simulink model "soft_finger_main"  (R2022b)
settings: Solver=VariableStepAuto  StartTime=0.0  StopTime=50  RelTol=1e-3
undefined symbols (not defined in the file): bounds, cf, D, DiscIntNeverNeededParam, Discrete, Fingertip, forceSetPoint, K, M, mylib, rho, sensor_locs, Time, X, Y, Z
libraries: sm_lib x117, nesl_utility x97, fl_lib x81, ee_lib x6, simulink x4, statsLibrary x3, slpidlib x2, deeplib x1, ctrlSharedLib x1
(part 2 of 5)

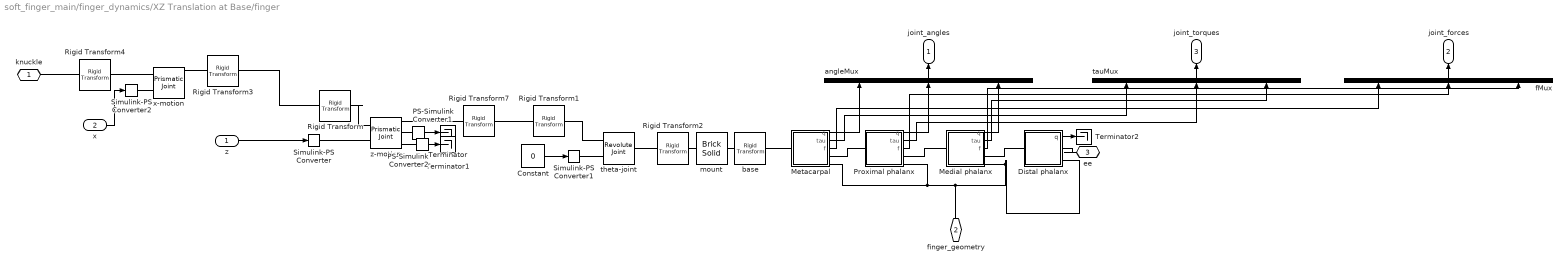
== system soft_finger_main/finger_dynamics/XZ Translation at Base/finger ==
  z : Inport
  x : Inport  Port=2
  Constant : Constant  Value=0
  Distal phalanx : Subsystem  mask{D=D, L=15, K=K, M=M, rho=rho, mu=1, muV=1}
  Medial phalanx : Subsystem  mask{D=D, L=24, K=K, M=M, rho=rho, mu=1, muV=1}
  Metacarpal : Subsystem  mask{D=D, L=64, K=K, M=M, rho=rho, mu=1, muV=1}
  PS-Simulink Converter1 : nesl_utility/PS-Simulink Converter  PhysicalDomain=network_engine_domain  SubClassName=ps_output  LeftPortType=input  RightPortType=output  PseudoPeriodic=off  Frequencies=[]  VectorFormat=1-D array  Unit=inherit  AffineConversion=off
  PS-Simulink Converter2 : nesl_utility/PS-Simulink Converter  PhysicalDomain=network_engine_domain  SubClassName=ps_output  LeftPortType=input  RightPortType=output  PseudoPeriodic=off  Frequencies=[]  VectorFormat=1-D array  Unit=inherit  AffineConversion=off
  Proximal phalanx : Subsystem  mask{D=D, L=39, K=K, M=M, rho=rho, mu=1, muV=1}
  Rigid Transform : sm_lib/Frames and Transforms/Rigid Transform  TranslationMethod=Cartesian  TranslationStandardOffset=40  TranslationLengthUnit=mm  TranslationStandardAxis=+Z  TranslationCartesianOffset=initPos  TranslationROffset=0  TranslationROffsetUnits=m  TranslationZOffset=0  TranslationZOffsetUnits=m  TranslationThetaOffset=0  TranslationThetaOffsetUnits=deg  RotationMethod=StandardAxis  RotationAngleUnits=deg  RotationStandardAxis=+Z  RotationAngle=180  RotationArbitraryAxis=[0 0 1]  FollAlignAxisA=+X  BaseAlignAxisA=+Y  FollAlignAxisB=+Y  BaseAlignAxisB=+Z  RotationSequenceAxes=FollowerAxes  RotationSequence=XYX  RotationSequenceAngles=[0 0 0]  RotationSequenceAnglesUnits=deg  RotationMatrix=[1 0 0; 0 1 0; 0 0 1]  Quaternion=[1 0 0 0]
  Rigid Transform1 : sm_lib/Frames and Transforms/Rigid Transform  TranslationMethod=None  TranslationStandardOffset=0  TranslationLengthUnit=m  TranslationStandardAxis=+Z  TranslationCartesianOffset=[0 0 0]  TranslationROffset=0  TranslationROffsetUnits=m  TranslationZOffset=0  TranslationZOffsetUnits=m  TranslationThetaOffset=0  TranslationThetaOffsetUnits=deg  RotationMethod=StandardAxis  RotationAngleUnits=deg  RotationStandardAxis=-X  RotationAngle=90  RotationArbitraryAxis=[0 0 1]  FollAlignAxisA=+X  BaseAlignAxisA=+Y  FollAlignAxisB=+Y  BaseAlignAxisB=+Z  RotationSequenceAxes=FollowerAxes  RotationSequence=XYX  RotationSequenceAngles=[0 0 0]  RotationSequenceAnglesUnits=deg  RotationMatrix=[1 0 0; 0 1 0; 0 0 1]  Quaternion=[1 0 0 0]
  Rigid Transform2 : sm_lib/Frames and Transforms/Rigid Transform  TranslationMethod=None  TranslationStandardOffset=0  TranslationLengthUnit=m  TranslationStandardAxis=+Z  TranslationCartesianOffset=[0 0 0]  TranslationROffset=0  TranslationROffsetUnits=m  TranslationZOffset=0  TranslationZOffsetUnits=m  TranslationThetaOffset=0  TranslationThetaOffsetUnits=deg  RotationMethod=StandardAxis  RotationAngleUnits=deg  RotationStandardAxis=-X  RotationAngle=90  RotationArbitraryAxis=[0 0 1]  FollAlignAxisA=+X  BaseAlignAxisA=+Y  FollAlignAxisB=+Y  BaseAlignAxisB=+Z  RotationSequenceAxes=FollowerAxes  RotationSequence=XYX  RotationSequenceAngles=[0 0 0]  RotationSequenceAnglesUnits=deg  RotationMatrix=[1 0 0; 0 1 0; 0 0 1]  Quaternion=[1 0 0 0]
  Rigid Transform3 : sm_lib/Frames and Transforms/Rigid Transform  TranslationMethod=None  TranslationStandardOffset=0  TranslationLengthUnit=m  TranslationStandardAxis=+Z  TranslationCartesianOffset=[0 0 0]  TranslationROffset=0  TranslationROffsetUnits=m  TranslationZOffset=0  TranslationZOffsetUnits=m  TranslationThetaOffset=0  TranslationThetaOffsetUnits=deg  RotationMethod=StandardAxis  RotationAngleUnits=deg  RotationStandardAxis=+Y  RotationAngle=90  RotationArbitraryAxis=[0 0 1]  FollAlignAxisA=+X  BaseAlignAxisA=+Y  FollAlignAxisB=+Y  BaseAlignAxisB=+Z  RotationSequenceAxes=FollowerAxes  RotationSequence=XYX  RotationSequenceAngles=[0 0 0]  RotationSequenceAnglesUnits=deg  RotationMatrix=[1 0 0; 0 1 0; 0 0 1]  Quaternion=[1 0 0 0]
  Rigid Transform4 : sm_lib/Frames and Transforms/Rigid Transform  TranslationMethod=None  TranslationStandardOffset=0  TranslationLengthUnit=m  TranslationStandardAxis=+Z  TranslationCartesianOffset=[0 0 0]  TranslationROffset=0  TranslationROffsetUnits=m  TranslationZOffset=0  TranslationZOffsetUnits=m  TranslationThetaOffset=0  TranslationThetaOffsetUnits=deg  RotationMethod=StandardAxis  RotationAngleUnits=deg  RotationStandardAxis=-Y  RotationAngle=90  RotationArbitraryAxis=[0 0 1]  FollAlignAxisA=+X  BaseAlignAxisA=+Y  FollAlignAxisB=+Y  BaseAlignAxisB=+Z  RotationSequenceAxes=FollowerAxes  RotationSequence=XYX  RotationSequenceAngles=[0 0 0]  RotationSequenceAnglesUnits=deg  RotationMatrix=[1 0 0; 0 1 0; 0 0 1]  Quaternion=[1 0 0 0]
  Rigid Transform7 : sm_lib/Frames and Transforms/Rigid Transform  TranslationMethod=None  TranslationStandardOffset=0  TranslationLengthUnit=m  TranslationStandardAxis=+Z  TranslationCartesianOffset=[0 0 0]  TranslationROffset=0  TranslationROffsetUnits=m  TranslationZOffset=0  TranslationZOffsetUnits=m  TranslationThetaOffset=0  TranslationThetaOffsetUnits=deg  RotationMethod=StandardAxis  RotationAngleUnits=rad  RotationStandardAxis=+Y  RotationAngle=0  RotationArbitraryAxis=[0 0 1]  FollAlignAxisA=+X  BaseAlignAxisA=+Y  FollAlignAxisB=+Y  BaseAlignAxisB=+Z  RotationSequenceAxes=FollowerAxes  RotationSequence=XYX  RotationSequenceAngles=[0 0 0]  RotationSequenceAnglesUnits=deg  RotationMatrix=[1 0 0; 0 1 0; 0 0 1]  Quaternion=[1 0 0 0]
  Simulink-PS Converter : nesl_utility/Simulink-PS Converter  PhysicalDomain=network_engine_domain  SubClassName=ps_input  LeftPortType=input  RightPortType=output  PseudoPeriodic=off  Frequencies=[]  NoiseDistribution=none  NoiseParameters=[]  Unit=mm  AffineConversion=off  FilteringAndDerivatives=filter  SimscapeFilterOrder=2  InputFilterTimeConstant=0.001  UdotUserProvided=0
  Simulink-PS Converter1 : nesl_utility/Simulink-PS Converter  PhysicalDomain=network_engine_domain  SubClassName=ps_input  LeftPortType=input  RightPortType=output  PseudoPeriodic=off  Frequencies=[]  NoiseDistribution=none  NoiseParameters=[]  Unit=rad  AffineConversion=off  FilteringAndDerivatives=filter  SimscapeFilterOrder=2  InputFilterTimeConstant=0.001  UdotUserProvided=0
  Simulink-PS Converter2 : nesl_utility/Simulink-PS Converter  PhysicalDomain=network_engine_domain  SubClassName=ps_input  LeftPortType=input  RightPortType=output  PseudoPeriodic=off  Frequencies=[]  NoiseDistribution=none  NoiseParameters=[]  Unit=mm  AffineConversion=off  FilteringAndDerivatives=filter  SimscapeFilterOrder=2  InputFilterTimeConstant=0.001  UdotUserProvided=0
  Terminator : Terminator
  Terminator1 : Terminator
  Terminator2 : Terminator
  angleMux : Mux  Inputs=3
  base : sm_lib/Frames and Transforms/Rigid Transform  TranslationMethod=None  TranslationStandardOffset=0  TranslationLengthUnit=m  TranslationStandardAxis=+Z  TranslationCartesianOffset=[0 0 0]  TranslationROffset=0  TranslationROffsetUnits=m  TranslationZOffset=0  TranslationZOffsetUnits=m  TranslationThetaOffset=0  TranslationThetaOffsetUnits=deg  RotationMethod=StandardAxis  RotationAngleUnits=deg  RotationStandardAxis=+Y  RotationAngle=90  RotationArbitraryAxis=[0 0 1]  FollAlignAxisA=+X  BaseAlignAxisA=+Y  FollAlignAxisB=+Y  BaseAlignAxisB=+Z  RotationSequenceAxes=FollowerAxes  RotationSequence=XYX  RotationSequenceAngles=[0 0 0]  RotationSequenceAnglesUnits=deg  RotationMatrix=[1 0 0; 0 1 0; 0 0 1]  Quaternion=[1 0 0 0]
  fMux : Mux  Inputs=3
  mount : sm_lib/Body Elements/Brick Solid  GraphicAmbientColor=[0.15 0.15 0.15 1.0]  BasedOnType=Density  BrickDimensions=[10 10 10]  BrickDimensionUnits=mm  CenterOfMass=[0 0 0]  CenterOfMassUnits=m  GraphicDiffuseColor=[.9 .9 1]  Density=1000  DensityUnits=kg/m^3  DoExposeReferenceFrame=on  GraphicEmissiveColor=[0.0 0.0 0.0 1.0]  ExportEntireGeometry=off  SerializedFrames=<Frames><Frame><Id>Frame1</Id><Value><Name>F1</Name><Origin><Source>GeometricFeature</Source><FeatureName>+x surface</FeatureName></Origin><PrimaryAxis><DefinedDirection>+Z</DefinedDirection><Source>ReferenceFrame</Source><SourceDirection>+Z</SourceDirection><FeatureName></FeatureName></PrimaryAxis><SecondaryAxis><DefinedDirection>+X</DefinedDirection><Source>ReferenceFrame</Source><SourceDirection>+X</SourceDirection><FeatureName></FeatureName></SecondaryAxis></Value></Frame></Frames>  MarkerShape=Sphere  MarkerSize=10  GraphicType=FromGeometry  InertiaType=CalculateFromGeometry  Mass=1  MassUnits=kg  MomentsOfInertia=[1 1 1]  MomentsOfInertiaUnits=kg*m^2  GraphicOpacity=1.0  ProductsOfInertia=[0 0 0]  ProductsOfInertiaUnits=kg*m^2  GraphicShininess=75  GraphicSpecularColor=[0.5 0.5 0.5 1.0]  GraphicVisPropType=SimpleVisualProperties
  tauMux : Mux  Inputs=3
  theta-joint : sm_lib/Joints/Revolute Joint  JointMode=Normal  SenseConstraintForce=off  SenseConstraintForceX=off  SenseConstraintForceY=off  SenseConstraintForceZ=off  SenseConstraintTorque=off  SenseConstraintTorqueX=off  SenseConstraintTorqueY=off  SenseConstraintTorqueZ=off  SenseTotalForce=off  SenseTotalForceX=off  SenseTotalForceY=off  SenseTotalForceZ=off  SenseTotalTorque=off  SenseTotalTorqueX=off  SenseTotalTorqueY=off  SenseTotalTorqueZ=off  CompositeWrenchDir=FollowerOnBase  CompositeWrenchFrame=BaseFrame  EquilibriumPosition=0  EquilibriumPositionUnits=deg  SpringStiffness=0  SpringStiffnessUnits=N*m/deg  DampingCoefficient=0  DampingCoefficientUnits=N*m/(deg/s)  TorqueActuationMode=ComputedTorque  MotionActuationMode=InputMotion  SensePosition=off  SenseVelocity=off  SenseAcceleration=off  SenseTorqueForce=off  SenseLowerLimitTorqueForce=off  SenseUpperLimitTorqueForce=off  LowerLimitSpecify=off  LowerLimitBound=-90  LowerLimitBoundUnits=deg  LowerLimitStiffness=1e4  LowerLimitStiffnessUnits=N*m/deg  LowerLimitDamping=10  LowerLimitDampingUnits=N*m/(deg/s)  LowerLimitTransitionRegionWidth=0.1  LowerLimitTransitionRegionWidthUnits=deg  UpperLimitSpecify=off  UpperLimitBound=90  UpperLimitBoundUnits=deg  UpperLimitStiffness=1e4  UpperLimitStiffnessUnits=N*m/deg  UpperLimitDamping=10  UpperLimitDampingUnits=N*m/(deg/s)  UpperLimitTransitionRegionWidth=0.1  UpperLimitTransitionRegionWidthUnits=deg  PositionTargetSpecify=off  PositionTargetPriority=High  PositionTargetValue=0  PositionTargetValueUnits=deg  VelocityTargetSpecify=off  VelocityTargetPriority=High  VelocityTargetValue=0  VelocityTargetValueUnits=deg/s
  x-motion : sm_lib/Joints/Prismatic Joint  JointMode=Normal  SenseConstraintForce=off  SenseConstraintForceX=off  SenseConstraintForceY=off  SenseConstraintForceZ=off  SenseConstraintTorque=off  SenseConstraintTorqueX=off  SenseConstraintTorqueY=off  SenseConstraintTorqueZ=off  SenseTotalForce=off  SenseTotalForceX=off  SenseTotalForceY=off  SenseTotalForceZ=off  SenseTotalTorque=off  SenseTotalTorqueX=off  SenseTotalTorqueY=off  SenseTotalTorqueZ=off  CompositeWrenchDir=FollowerOnBase  CompositeWrenchFrame=BaseFrame  EquilibriumPosition=0  EquilibriumPositionUnits=m  SpringStiffness=0  SpringStiffnessUnits=N/m  DampingCoefficient=0  DampingCoefficientUnits=N/(m/s)  TorqueActuationMode=ComputedTorque  MotionActuationMode=InputMotion  SensePosition=on  SenseVelocity=off  SenseAcceleration=off  SenseTorqueForce=on  SenseLowerLimitTorqueForce=off  SenseUpperLimitTorqueForce=off  LowerLimitSpecify=off  LowerLimitBound=-1  LowerLimitBoundUnits=m  LowerLimitStiffness=1e6  LowerLimitStiffnessUnits=N/m  LowerLimitDamping=1e3  LowerLimitDampingUnits=N/(m/s)  LowerLimitTransitionRegionWidth=1e-4  LowerLimitTransitionRegionWidthUnits=m  UpperLimitSpecify=off  UpperLimitBound=1  UpperLimitBoundUnits=m  UpperLimitStiffness=1e6  UpperLimitStiffnessUnits=N/m  UpperLimitDamping=1e3  UpperLimitDampingUnits=N/(m/s)  UpperLimitTransitionRegionWidth=1e-4  UpperLimitTransitionRegionWidthUnits=m  PositionTargetSpecify=off  PositionTargetPriority=High  PositionTargetValue=0  PositionTargetValueUnits=m  VelocityTargetSpecify=off  VelocityTargetPriority=High  VelocityTargetValue=0  VelocityTargetValueUnits=m/s
  z-motion : sm_lib/Joints/Prismatic Joint  JointMode=Normal  SenseConstraintForce=off  SenseConstraintForceX=off  SenseConstraintForceY=off  SenseConstraintForceZ=off  SenseConstraintTorque=off  SenseConstraintTorqueX=off  SenseConstraintTorqueY=off  SenseConstraintTorqueZ=off  SenseTotalForce=off  SenseTotalForceX=off  SenseTotalForceY=off  SenseTotalForceZ=off  SenseTotalTorque=off  SenseTotalTorqueX=off  SenseTotalTorqueY=off  SenseTotalTorqueZ=off  CompositeWrenchDir=FollowerOnBase  CompositeWrenchFrame=BaseFrame  EquilibriumPosition=0  EquilibriumPositionUnits=m  SpringStiffness=0  SpringStiffnessUnits=N/m  DampingCoefficient=0  DampingCoefficientUnits=N/(m/s)  TorqueActuationMode=ComputedTorque  MotionActuationMode=InputMotion  SensePosition=on  SenseVelocity=off  SenseAcceleration=off  SenseTorqueForce=on  SenseLowerLimitTorqueForce=off  SenseUpperLimitTorqueForce=off  LowerLimitSpecify=off  LowerLimitBound=-1  LowerLimitBoundUnits=m  LowerLimitStiffness=1e6  LowerLimitStiffnessUnits=N/m  LowerLimitDamping=1e3  LowerLimitDampingUnits=N/(m/s)  LowerLimitTransitionRegionWidth=1e-4  LowerLimitTransitionRegionWidthUnits=m  UpperLimitSpecify=off  UpperLimitBound=1  UpperLimitBoundUnits=m  UpperLimitStiffness=1e6  UpperLimitStiffnessUnits=N/m  UpperLimitDamping=1e3  UpperLimitDampingUnits=N/(m/s)  UpperLimitTransitionRegionWidth=1e-4  UpperLimitTransitionRegionWidthUnits=m  PositionTargetSpecify=off  PositionTargetPriority=High  PositionTargetValue=0  PositionTargetValueUnits=m  VelocityTargetSpecify=off  VelocityTargetPriority=High  VelocityTargetValue=0  VelocityTargetValueUnits=m/s
  knuckle : PMIOPort  Side=Left
  finger_geometry : PMIOPort  Port=2  Side=Left
  ee : PMIOPort  Port=3  Side=Right
  joint_angles : Outport
  joint_forces : Outport  Port=2
  joint_torques : Outport  Port=3
  wires:
  z/1 -> Simulink-PS Converter/1
  PS-Simulink Converter1/1 -> Terminator/1
  PS-Simulink Converter2/1 -> Terminator1/1
  x/1 -> Simulink-PS Converter2/1
  Proximal phalanx/3(f) -> fMux/2
  Metacarpal/2(tau) -> tauMux/1
  Medial phalanx/3(f) -> fMux/3
  Medial phalanx/2(tau) -> tauMux/3
  tauMux/1 -> joint_torques/1
  Metacarpal/1(q) -> angleMux/1
  Medial phalanx/1(q) -> angleMux/3
  angleMux/1 -> joint_angles/1
  Metacarpal/3(f) -> fMux/1
  Proximal phalanx/2(tau) -> tauMux/2
  Distal phalanx/1(q) -> Terminator2/1
  Proximal phalanx/1(q) -> angleMux/2
  fMux/1 -> joint_forces/1
  Constant/1 -> Simulink-PS Converter1/1
  connections:
  Simulink-PS Converter1/RConn1 -- theta-joint/LConn2
  Simulink-PS Converter/RConn1 -- z-motion/LConn2
  z-motion/RConn1 -- Rigid Transform7/LConn1
  Rigid Transform2/LConn1 -- mount/RConn1
  Rigid Transform1/RConn1 -- theta-joint/LConn1
  Rigid Transform7/RConn1 -- Rigid Transform1/LConn1
  theta-joint/RConn1 -- Rigid Transform2/RConn1
  Rigid Transform/RConn1 -- z-motion/LConn1
  mount/LConn1 -- base/LConn1
  Rigid Transform/LConn1 -- Rigid Transform3/RConn1
  z-motion/RConn2 -- PS-Simulink Converter1/LConn1
  z-motion/RConn3 -- PS-Simulink Converter2/LConn1
  Rigid Transform3/LConn1 -- x-motion/RConn1
  x-motion/LConn1 -- Rigid Transform4/RConn1
  Simulink-PS Converter2/RConn1 -- x-motion/LConn2
  Rigid Transform4/LConn1 -- knuckle/RConn1
  Medial phalanx/RConn2 -- Distal phalanx/RConn2 -- Metacarpal/RConn2 -- Proximal phalanx/RConn2 -- finger_geometry/RConn1
  Metacarpal/RConn1 -- Proximal phalanx/LConn1
  Medial phalanx/LConn1 -- Proximal phalanx/RConn1
  ee/RConn1 -- Distal phalanx/RConn1
  Medial phalanx/RConn1 -- Distal phalanx/LConn1
  base/RConn1 -- Metacarpal/LConn1

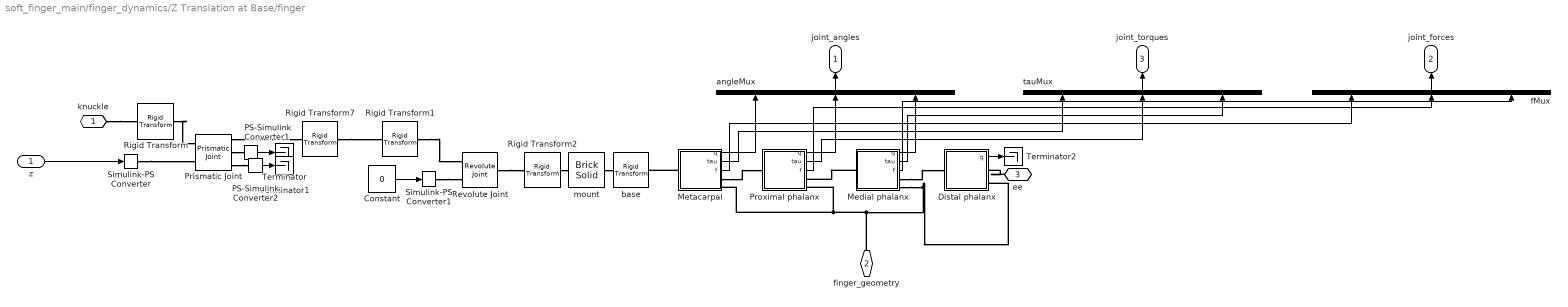
== system soft_finger_main/finger_dynamics/Z Translation at Base/finger ==
  z : Inport
  Constant : Constant  Value=0
  Distal phalanx : Subsystem  mask{D=D, L=15, K=K, M=M, rho=rho, mu=1, muV=1}
  Medial phalanx : Subsystem  mask{D=D, L=24, K=K, M=M, rho=rho, mu=1, muV=1}
  Metacarpal : Subsystem  mask{D=D, L=64, K=K, M=M, rho=rho, mu=1, muV=1}
  PS-Simulink Converter1 : nesl_utility/PS-Simulink Converter  PhysicalDomain=network_engine_domain  SubClassName=ps_output  LeftPortType=input  RightPortType=output  PseudoPeriodic=off  Frequencies=[]  VectorFormat=1-D array  Unit=inherit  AffineConversion=off
  PS-Simulink Converter2 : nesl_utility/PS-Simulink Converter  PhysicalDomain=network_engine_domain  SubClassName=ps_output  LeftPortType=input  RightPortType=output  PseudoPeriodic=off  Frequencies=[]  VectorFormat=1-D array  Unit=inherit  AffineConversion=off
  Prismatic Joint : sm_lib/Joints/Prismatic Joint  JointMode=Normal  SenseConstraintForce=off  SenseConstraintForceX=off  SenseConstraintForceY=off  SenseConstraintForceZ=off  SenseConstraintTorque=off  SenseConstraintTorqueX=off  SenseConstraintTorqueY=off  SenseConstraintTorqueZ=off  SenseTotalForce=off  SenseTotalForceX=off  SenseTotalForceY=off  SenseTotalForceZ=off  SenseTotalTorque=off  SenseTotalTorqueX=off  SenseTotalTorqueY=off  SenseTotalTorqueZ=off  CompositeWrenchDir=FollowerOnBase  CompositeWrenchFrame=BaseFrame  EquilibriumPosition=0  EquilibriumPositionUnits=m  SpringStiffness=0  SpringStiffnessUnits=N/m  DampingCoefficient=0  DampingCoefficientUnits=N/(m/s)  TorqueActuationMode=ComputedTorque  MotionActuationMode=InputMotion  SensePosition=on  SenseVelocity=off  SenseAcceleration=off  SenseTorqueForce=on  SenseLowerLimitTorqueForce=off  SenseUpperLimitTorqueForce=off  LowerLimitSpecify=off  LowerLimitBound=-1  LowerLimitBoundUnits=m  LowerLimitStiffness=1e6  LowerLimitStiffnessUnits=N/m  LowerLimitDamping=1e3  LowerLimitDampingUnits=N/(m/s)  LowerLimitTransitionRegionWidth=1e-4  LowerLimitTransitionRegionWidthUnits=m  UpperLimitSpecify=off  UpperLimitBound=1  UpperLimitBoundUnits=m  UpperLimitStiffness=1e6  UpperLimitStiffnessUnits=N/m  UpperLimitDamping=1e3  UpperLimitDampingUnits=N/(m/s)  UpperLimitTransitionRegionWidth=1e-4  UpperLimitTransitionRegionWidthUnits=m  PositionTargetSpecify=off  PositionTargetPriority=High  PositionTargetValue=0  PositionTargetValueUnits=m  VelocityTargetSpecify=off  VelocityTargetPriority=High  VelocityTargetValue=0  VelocityTargetValueUnits=m/s
  Proximal phalanx : Subsystem  mask{D=D, L=39, K=K, M=M, rho=rho, mu=1, muV=1}
  Revolute Joint : sm_lib/Joints/Revolute Joint  JointMode=Normal  SenseConstraintForce=off  SenseConstraintForceX=off  SenseConstraintForceY=off  SenseConstraintForceZ=off  SenseConstraintTorque=off  SenseConstraintTorqueX=off  SenseConstraintTorqueY=off  SenseConstraintTorqueZ=off  SenseTotalForce=off  SenseTotalForceX=off  SenseTotalForceY=off  SenseTotalForceZ=off  SenseTotalTorque=off  SenseTotalTorqueX=off  SenseTotalTorqueY=off  SenseTotalTorqueZ=off  CompositeWrenchDir=FollowerOnBase  CompositeWrenchFrame=BaseFrame  EquilibriumPosition=0  EquilibriumPositionUnits=deg  SpringStiffness=0  SpringStiffnessUnits=N*m/deg  DampingCoefficient=0  DampingCoefficientUnits=N*m/(deg/s)  TorqueActuationMode=ComputedTorque  MotionActuationMode=InputMotion  SensePosition=off  SenseVelocity=off  SenseAcceleration=off  SenseTorqueForce=off  SenseLowerLimitTorqueForce=off  SenseUpperLimitTorqueForce=off  LowerLimitSpecify=off  LowerLimitBound=-90  LowerLimitBoundUnits=deg  LowerLimitStiffness=1e4  LowerLimitStiffnessUnits=N*m/deg  LowerLimitDamping=10  LowerLimitDampingUnits=N*m/(deg/s)  LowerLimitTransitionRegionWidth=0.1  LowerLimitTransitionRegionWidthUnits=deg  UpperLimitSpecify=off  UpperLimitBound=90  UpperLimitBoundUnits=deg  UpperLimitStiffness=1e4  UpperLimitStiffnessUnits=N*m/deg  UpperLimitDamping=10  UpperLimitDampingUnits=N*m/(deg/s)  UpperLimitTransitionRegionWidth=0.1  UpperLimitTransitionRegionWidthUnits=deg  PositionTargetSpecify=off  PositionTargetPriority=High  PositionTargetValue=0  PositionTargetValueUnits=deg  VelocityTargetSpecify=off  VelocityTargetPriority=High  VelocityTargetValue=0  VelocityTargetValueUnits=deg/s
  Rigid Transform : sm_lib/Frames and Transforms/Rigid Transform  TranslationMethod=Cartesian  TranslationStandardOffset=40  TranslationLengthUnit=mm  TranslationStandardAxis=+Z  TranslationCartesianOffset=initPos  TranslationROffset=0  TranslationROffsetUnits=m  TranslationZOffset=0  TranslationZOffsetUnits=m  TranslationThetaOffset=0  TranslationThetaOffsetUnits=deg  RotationMethod=StandardAxis  RotationAngleUnits=deg  RotationStandardAxis=+Z  RotationAngle=180  RotationArbitraryAxis=[0 0 1]  FollAlignAxisA=+X  BaseAlignAxisA=+Y  FollAlignAxisB=+Y  BaseAlignAxisB=+Z  RotationSequenceAxes=FollowerAxes  RotationSequence=XYX  RotationSequenceAngles=[0 0 0]  RotationSequenceAnglesUnits=deg  RotationMatrix=[1 0 0; 0 1 0; 0 0 1]  Quaternion=[1 0 0 0]
  Rigid Transform1 : sm_lib/Frames and Transforms/Rigid Transform  TranslationMethod=None  TranslationStandardOffset=0  TranslationLengthUnit=m  TranslationStandardAxis=+Z  TranslationCartesianOffset=[0 0 0]  TranslationROffset=0  TranslationROffsetUnits=m  TranslationZOffset=0  TranslationZOffsetUnits=m  TranslationThetaOffset=0  TranslationThetaOffsetUnits=deg  RotationMethod=StandardAxis  RotationAngleUnits=deg  RotationStandardAxis=-X  RotationAngle=90  RotationArbitraryAxis=[0 0 1]  FollAlignAxisA=+X  BaseAlignAxisA=+Y  FollAlignAxisB=+Y  BaseAlignAxisB=+Z  RotationSequenceAxes=FollowerAxes  RotationSequence=XYX  RotationSequenceAngles=[0 0 0]  RotationSequenceAnglesUnits=deg  RotationMatrix=[1 0 0; 0 1 0; 0 0 1]  Quaternion=[1 0 0 0]
  Rigid Transform2 : sm_lib/Frames and Transforms/Rigid Transform  TranslationMethod=None  TranslationStandardOffset=0  TranslationLengthUnit=m  TranslationStandardAxis=+Z  TranslationCartesianOffset=[0 0 0]  TranslationROffset=0  TranslationROffsetUnits=m  TranslationZOffset=0  TranslationZOffsetUnits=m  TranslationThetaOffset=0  TranslationThetaOffsetUnits=deg  RotationMethod=StandardAxis  RotationAngleUnits=deg  RotationStandardAxis=-X  RotationAngle=90  RotationArbitraryAxis=[0 0 1]  FollAlignAxisA=+X  BaseAlignAxisA=+Y  FollAlignAxisB=+Y  BaseAlignAxisB=+Z  RotationSequenceAxes=FollowerAxes  RotationSequence=XYX  RotationSequenceAngles=[0 0 0]  RotationSequenceAnglesUnits=deg  RotationMatrix=[1 0 0; 0 1 0; 0 0 1]  Quaternion=[1 0 0 0]
  Rigid Transform7 : sm_lib/Frames and Transforms/Rigid Transform  TranslationMethod=None  TranslationStandardOffset=0  TranslationLengthUnit=m  TranslationStandardAxis=+Z  TranslationCartesianOffset=[0 0 0]  TranslationROffset=0  TranslationROffsetUnits=m  TranslationZOffset=0  TranslationZOffsetUnits=m  TranslationThetaOffset=0  TranslationThetaOffsetUnits=deg  RotationMethod=StandardAxis  RotationAngleUnits=rad  RotationStandardAxis=+Y  RotationAngle=0  RotationArbitraryAxis=[0 0 1]  FollAlignAxisA=+X  BaseAlignAxisA=+Y  FollAlignAxisB=+Y  BaseAlignAxisB=+Z  RotationSequenceAxes=FollowerAxes  RotationSequence=XYX  RotationSequenceAngles=[0 0 0]  RotationSequenceAnglesUnits=deg  RotationMatrix=[1 0 0; 0 1 0; 0 0 1]  Quaternion=[1 0 0 0]
  Simulink-PS Converter : nesl_utility/Simulink-PS Converter  PhysicalDomain=network_engine_domain  SubClassName=ps_input  LeftPortType=input  RightPortType=output  PseudoPeriodic=off  Frequencies=[]  NoiseDistribution=none  NoiseParameters=[]  Unit=mm  AffineConversion=off  FilteringAndDerivatives=filter  SimscapeFilterOrder=2  InputFilterTimeConstant=0.001  UdotUserProvided=0
  Simulink-PS Converter1 : nesl_utility/Simulink-PS Converter  PhysicalDomain=network_engine_domain  SubClassName=ps_input  LeftPortType=input  RightPortType=output  PseudoPeriodic=off  Frequencies=[]  NoiseDistribution=none  NoiseParameters=[]  Unit=rad  AffineConversion=off  FilteringAndDerivatives=filter  SimscapeFilterOrder=2  InputFilterTimeConstant=0.001  UdotUserProvided=0
  Terminator : Terminator
  Terminator1 : Terminator
  Terminator2 : Terminator
  angleMux : Mux  Inputs=3
  base : sm_lib/Frames and Transforms/Rigid Transform  TranslationMethod=None  TranslationStandardOffset=0  TranslationLengthUnit=m  TranslationStandardAxis=+Z  TranslationCartesianOffset=[0 0 0]  TranslationROffset=0  TranslationROffsetUnits=m  TranslationZOffset=0  TranslationZOffsetUnits=m  TranslationThetaOffset=0  TranslationThetaOffsetUnits=deg  RotationMethod=StandardAxis  RotationAngleUnits=deg  RotationStandardAxis=+Y  RotationAngle=90  RotationArbitraryAxis=[0 0 1]  FollAlignAxisA=+X  BaseAlignAxisA=+Y  FollAlignAxisB=+Y  BaseAlignAxisB=+Z  RotationSequenceAxes=FollowerAxes  RotationSequence=XYX  RotationSequenceAngles=[0 0 0]  RotationSequenceAnglesUnits=deg  RotationMatrix=[1 0 0; 0 1 0; 0 0 1]  Quaternion=[1 0 0 0]
  fMux : Mux  Inputs=3
  mount : sm_lib/Body Elements/Brick Solid  GraphicAmbientColor=[0.15 0.15 0.15 1.0]  BasedOnType=Density  BrickDimensions=[10 10 10]  BrickDimensionUnits=mm  CenterOfMass=[0 0 0]  CenterOfMassUnits=m  GraphicDiffuseColor=[.9 .9 1]  Density=1000  DensityUnits=kg/m^3  DoExposeReferenceFrame=on  GraphicEmissiveColor=[0.0 0.0 0.0 1.0]  ExportEntireGeometry=off  SerializedFrames=<Frames><Frame><Id>Frame1</Id><Value><Name>F1</Name><Origin><Source>GeometricFeature</Source><FeatureName>+x surface</FeatureName></Origin><PrimaryAxis><DefinedDirection>+Z</DefinedDirection><Source>ReferenceFrame</Source><SourceDirection>+Z</SourceDirection><FeatureName></FeatureName></PrimaryAxis><SecondaryAxis><DefinedDirection>+X</DefinedDirection><Source>ReferenceFrame</Source><SourceDirection>+X</SourceDirection><FeatureName></FeatureName></SecondaryAxis></Value></Frame></Frames>  MarkerShape=Sphere  MarkerSize=10  GraphicType=FromGeometry  InertiaType=CalculateFromGeometry  Mass=1  MassUnits=kg  MomentsOfInertia=[1 1 1]  MomentsOfInertiaUnits=kg*m^2  GraphicOpacity=1.0  ProductsOfInertia=[0 0 0]  ProductsOfInertiaUnits=kg*m^2  GraphicShininess=75  GraphicSpecularColor=[0.5 0.5 0.5 1.0]  GraphicVisPropType=SimpleVisualProperties
  tauMux : Mux  Inputs=3
  knuckle : PMIOPort  Side=Left
  finger_geometry : PMIOPort  Port=2  Side=Left
  ee : PMIOPort  Port=3  Side=Right
  joint_angles : Outport
  joint_forces : Outport  Port=2
  joint_torques : Outport  Port=3
  wires:
  Constant/1 -> Simulink-PS Converter1/1
  Proximal phalanx/1(q) -> angleMux/2
  Metacarpal/1(q) -> angleMux/1
  Medial phalanx/1(q) -> angleMux/3
  angleMux/1 -> joint_angles/1
  z/1 -> Simulink-PS Converter/1
  PS-Simulink Converter1/1 -> Terminator/1
  PS-Simulink Converter2/1 -> Terminator1/1
  Distal phalanx/1(q) -> Terminator2/1
  Proximal phalanx/2(tau) -> tauMux/2
  Medial phalanx/2(tau) -> tauMux/3
  tauMux/1 -> joint_torques/1
  fMux/1 -> joint_forces/1
  Metacarpal/2(tau) -> tauMux/1
  Metacarpal/3(f) -> fMux/1
  Proximal phalanx/3(f) -> fMux/2
  Medial phalanx/3(f) -> fMux/3
  connections:
  Medial phalanx/LConn1 -- Proximal phalanx/RConn1
  Simulink-PS Converter1/RConn1 -- Revolute Joint/LConn2
  Simulink-PS Converter/RConn1 -- Prismatic Joint/LConn2
  Prismatic Joint/RConn1 -- Rigid Transform7/LConn1
  Rigid Transform2/LConn1 -- mount/RConn1
  Rigid Transform1/RConn1 -- Revolute Joint/LConn1
  Rigid Transform7/RConn1 -- Rigid Transform1/LConn1
  Revolute Joint/RConn1 -- Rigid Transform2/RConn1
  Rigid Transform/RConn1 -- Prismatic Joint/LConn1
  mount/LConn1 -- base/LConn1
  Metacarpal/RConn2 -- Proximal phalanx/RConn2 -- finger_geometry/RConn1 -- Distal phalanx/RConn2 -- Medial phalanx/RConn2
  knuckle/RConn1 -- Rigid Transform/LConn1
  Metacarpal/RConn1 -- Proximal phalanx/LConn1
  Metacarpal/LConn1 -- base/RConn1
  Medial phalanx/RConn1 -- Distal phalanx/LConn1
  ee/RConn1 -- Distal phalanx/RConn1
  Prismatic Joint/RConn2 -- PS-Simulink Converter1/LConn1
  Prismatic Joint/RConn3 -- PS-Simulink Converter2/LConn1

== system soft_finger_main/platform/long_platform/platform ==
  GT sensor platform : sm_lib/Body Elements/Brick Solid  GraphicAmbientColor=[0.15 0.15 0.15 1.0]  BasedOnType=Density  BrickDimensions=[1000 300 10]  BrickDimensionUnits=mm  CenterOfMass=[0 0 0]  CenterOfMassUnits=m  GraphicDiffuseColor=[.1 .1 .1]  Density=50  DensityUnits=kg/m^3  DoExposeReferenceFrame=off  GraphicEmissiveColor=[0.0 0.0 0.0 1.0]  ExportEntireGeometry=on  SerializedFrames=<Frames><Frame><Id>Frame1</Id><Value><Name>R</Name><Origin><Source>CenterOfMassFrame</Source><FeatureName></FeatureName></Origin><PrimaryAxis><DefinedDirection>+Z</DefinedDirection><Source>ReferenceFrame</Source><SourceDirection>+Z</SourceDirection><FeatureName></FeatureName></PrimaryAxis><SecondaryAxis><DefinedDirection>+X</DefinedDirection><Source>ReferenceFrame</Source><SourceDirection>+X</SourceDirection><FeatureName></FeatureName></SecondaryAxis></Value></Frame><Frame><Id>Frame2</Id><Value><Name>F2</Name><Origin><Source>GeometricFeature</Source><FeatureName>+z surface</FeatureName></Origin><PrimaryAxis><DefinedDirection>+Z</DefinedDirection><Source>ReferenceFrame</Source><SourceDirection>+Z</SourceDirection><FeatureName></FeatureName></PrimaryAxis><SecondaryAxis><DefinedDirection>+X</DefinedDirection><Source>ReferenceFrame</Source><SourceDirection>+X</SourceDirection><FeatureName></FeatureName></SecondaryAxis></Value></Frame></Frames>  MarkerShape=Sphere  MarkerSize=10  GraphicType=FromGeometry  InertiaType=CalculateFromGeometry  Mass=1  MassUnits=kg  MomentsOfInertia=[1 1 1]  MomentsOfInertiaUnits=kg*m^2  GraphicOpacity=0.1  ProductsOfInertia=[0 0 0]  ProductsOfInertiaUnits=kg*m^2  GraphicShininess=75  GraphicSpecularColor=[0.5 0.5 0.5 1.0]  GraphicVisPropType=SimpleVisualProperties
  PS-Simulink Converter : nesl_utility/PS-Simulink Converter  PhysicalDomain=network_engine_domain  SubClassName=ps_output  LeftPortType=input  RightPortType=output  PseudoPeriodic=off  Frequencies=[]  VectorFormat=1-D array  Unit=inherit  AffineConversion=off
  Rate Transition1 : RateTransition  InitialCondition=0;  OutPortSampleTime=1/cf;
  Rate Transition2 : RateTransition  InitialCondition=0;  OutPortSampleTime=1/cf;
  Rate Transition3 : RateTransition  InitialCondition=0;  OutPortSampleTime=1/cf;
  Sensor : sm_lib/Frames and Transforms/Transform Sensor  MeasurementFrame=World  SenseAngle=off  SenseAxis=off  SenseQ=off  SenseR=off  SenseRotationSequence=off  RotationSequence=XYX  SenseOmegaX=off  SenseOmegaY=off  SenseOmegaZ=off  SenseQDot=off  SenseRDot=off  SenseAlphaX=off  SenseAlphaY=off  SenseAlphaZ=off  SenseQDDot=off  SenseRDDot=off  SenseX=off  SenseY=off  SenseZ=on  SenseRad=off  SenseAzim=off  SenseDist=off  SenseInc=off  SenseXDot=off  SenseYDot=off  SenseZDot=off  SenseRadDot=off  SenseAzimDot=off  SenseDistDot=off  SenseIncDot=off  SenseXDDot=off  SenseYDDot=off  SenseZDDot=off  SenseRadDDot=off  SenseAzimDDot=off  SenseDistDDot=off  SenseIncDDot=off
  Terminator : Terminator
  finger_tip : Subsystem  Variant=on  VariantControlMode=label  VariantControl=Choice  LabelModeActiveChoice=sphere
  platform_geometry : PMIOPort  Side=Left
  platform_R : PMIOPort  Port=2  Side=Left
  platform_F2 : PMIOPort  Port=3  Side=Right
  normal_force : Outport
  friction_force : Outport  Port=2
  separation_distance : Outport  Port=3
  wires:
  PS-Simulink Converter/1 -> Terminator/1
  Rate Transition2/1 -> normal_force/1
  Rate Transition1/1 -> friction_force/1
  Rate Transition3/1 -> separation_distance/1
  finger_tip/1(Normal force) -> Rate Transition2/1
  finger_tip/2(Friction force) -> Rate Transition1/1
  finger_tip/3(separation distance) -> Rate Transition3/1
  connections:
  GT sensor platform/RConn1 -- Sensor/LConn1
  Sensor/RConn2 -- PS-Simulink Converter/LConn1
  platform_R/RConn1 -- GT sensor platform/LConn1
  platform_F2/RConn1 -- Sensor/RConn1 -- finger_tip/LConn1
  platform_geometry/RConn1 -- GT sensor platform/LConn2 -- finger_tip/RConn1

== system soft_finger_main/platform/short_platform/platform ==
  GT sensor platform : sm_lib/Body Elements/Brick Solid  GraphicAmbientColor=[0.15 0.15 0.15 1.0]  BasedOnType=Density  BrickDimensions=[100 100 10]  BrickDimensionUnits=mm  CenterOfMass=[0 0 0]  CenterOfMassUnits=m  GraphicDiffuseColor=[.1 .1 .1]  Density=50  DensityUnits=kg/m^3  DoExposeReferenceFrame=off  GraphicEmissiveColor=[0.0 0.0 0.0 1.0]  ExportEntireGeometry=on  SerializedFrames=<Frames><Frame><Id>Frame1</Id><Value><Name>F1</Name><Origin><Source>GeometricFeature</Source><FeatureName>-x surface</FeatureName></Origin><PrimaryAxis><DefinedDirection>+Z</DefinedDirection><Source>ReferenceFrame</Source><SourceDirection>+Z</SourceDirection><FeatureName></FeatureName></PrimaryAxis><SecondaryAxis><DefinedDirection>+X</DefinedDirection><Source>ReferenceFrame</Source><SourceDirection>+X</SourceDirection><FeatureName></FeatureName></SecondaryAxis></Value></Frame><Frame><Id>Frame2</Id><Value><Name>F2</Name><Origin><Source>GeometricFeature</Source><FeatureName>+z surface</FeatureName></Origin><PrimaryAxis><DefinedDirection>+Z</DefinedDirection><Source>ReferenceFrame</Source><SourceDirection>+Z</SourceDirection><FeatureName></FeatureName></PrimaryAxis><SecondaryAxis><DefinedDirection>+X</DefinedDirection><Source>ReferenceFrame</Source><SourceDirection>+X</SourceDirection><FeatureName></FeatureName></SecondaryAxis></Value></Frame></Frames>  MarkerShape=Sphere  MarkerSize=10  GraphicType=FromGeometry  InertiaType=CalculateFromGeometry  Mass=1  MassUnits=kg  MomentsOfInertia=[1 1 1]  MomentsOfInertiaUnits=kg*m^2  GraphicOpacity=1.0  ProductsOfInertia=[0 0 0]  ProductsOfInertiaUnits=kg*m^2  GraphicShininess=75  GraphicSpecularColor=[0.5 0.5 0.5 1.0]  GraphicVisPropType=SimpleVisualProperties
  PS-Simulink Converter : nesl_utility/PS-Simulink Converter  PhysicalDomain=network_engine_domain  SubClassName=ps_output  LeftPortType=input  RightPortType=output  PseudoPeriodic=off  Frequencies=[]  VectorFormat=1-D array  Unit=inherit  AffineConversion=off
  Rate Transition2 : RateTransition  InitialCondition=0;  OutPortSampleTime=1/cf;
  Sensor : sm_lib/Frames and Transforms/Transform Sensor  MeasurementFrame=World  SenseAngle=off  SenseAxis=off  SenseQ=off  SenseR=off  SenseRotationSequence=off  RotationSequence=XYX  SenseOmegaX=off  SenseOmegaY=off  SenseOmegaZ=off  SenseQDot=off  SenseRDot=off  SenseAlphaX=off  SenseAlphaY=off  SenseAlphaZ=off  SenseQDDot=off  SenseRDDot=off  SenseX=off  SenseY=off  SenseZ=on  SenseRad=off  SenseAzim=off  SenseDist=off  SenseInc=off  SenseXDot=off  SenseYDot=off  SenseZDot=off  SenseRadDot=off  SenseAzimDot=off  SenseDistDot=off  SenseIncDot=off  SenseXDDot=off  SenseYDDot=off  SenseZDDot=off  SenseRadDDot=off  SenseAzimDDot=off  SenseDistDDot=off  SenseIncDDot=off
  Terminator : Terminator
  finger_tip : Subsystem  AncestorBlock=mylib/Fingertip  mask{D=D, rho=rho, mu=1, muV=1}
      mask prompts: D "Diameter"
      settings: LibrarySourceBlock=mylib/Fingertip
  platform_geometry : PMIOPort  Side=Left
  platform_F1 : PMIOPort  Port=2  Side=Left
  platform_F2 : PMIOPort  Port=3  Side=Right
  normal_force : Outport
  wires:
  finger_tip/1(Normal force) -> Rate Transition2/1
  PS-Simulink Converter/1 -> Terminator/1
  Rate Transition2/1 -> normal_force/1
  connections:
  finger_tip/RConn1 -- GT sensor platform/LConn2 -- platform_geometry/RConn1
  GT sensor platform/RConn1 -- Sensor/LConn1
  Sensor/RConn1 -- finger_tip/LConn1 -- platform_F2/RConn1
  Sensor/RConn2 -- PS-Simulink Converter/LConn1
  platform_F1/RConn1 -- GT sensor platform/LConn1

== system soft_finger_main/state_estimation/custom/friction_state_estimator ==
  In1 : Inport
  Constant : Constant  Value=0
  Terminator : Terminator
  Out1 : Outport
  wires:
  In1/1 -> Terminator/1
  Constant/1 -> Out1/1

== system soft_finger_main/state_estimation/custom/normal_force_state_estimator ==
  In1 : Inport
  Constant : Constant  Value=0
  Terminator : Terminator
  Out1 : Outport
  wires:
  Constant/1 -> Out1/1
  In1/1 -> Terminator/1

== system soft_finger_main/state_estimation/off/friction_state_estimator ==
  In1 : Inport
  Constant : Constant  Value=0
  Terminator : Terminator
  Out1 : Outport
  wires:
  Constant/1 -> Out1/1
  In1/1 -> Terminator/1

== system soft_finger_main/state_estimation/off/normal_force_state_estimator ==
  In1 : Inport
  Constant : Constant  Value=0
  Terminator : Terminator
  Out1 : Outport
  wires:
  In1/1 -> Terminator/1
  Constant/1 -> Out1/1

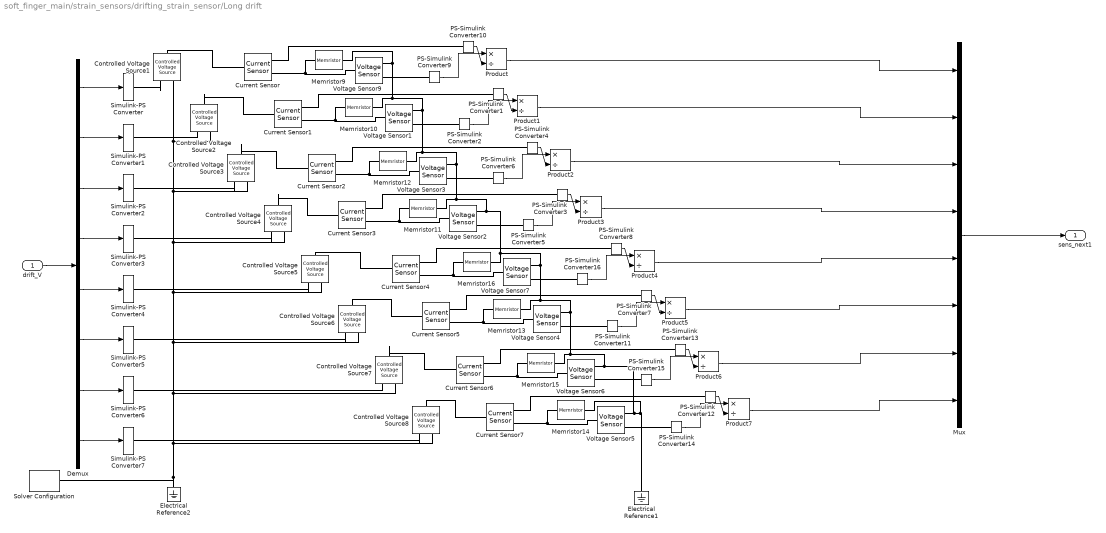
== system soft_finger_main/strain_sensors/drifting_strain_sensor/Long drift ==
  drift_V : Inport
  Controlled Voltage Source{1..8} (8 alike) : fl_lib/Electrical/Electrical Sources/Controlled Voltage Source
  Current Sensor{,1..7} (8 alike) : fl_lib/Electrical/Electrical Sensors/Current Sensor
  Demux : Demux  Outputs=8
  Electrical Reference1 : fl_lib/Electrical/Electrical Elements/Electrical Reference
  Electrical Reference2 : fl_lib/Electrical/Electrical Elements/Electrical Reference
  Memristor10 : fl_lib/Electrical/Electrical Elements/Memristor  Ra=10500 Ohm  Rb=9500 Ohm  Q0=1.45e-2 C  x0=0.2  pwindow=2  i_specify=off  i_priority=None  i=0 A  i_nominal_specify=off  i_nominal_unit=A  i_nominal_value=1  v_specify=off  v_priority=None  v=0 V  v_nominal_specify=off  v_nominal_unit=V  v_nominal_value=1
      settings: InternalSimscapePortConfiguration="{\"Bottom\":[],\"Left\":[{\"id\":\"p\",\"label\":\"+\",\"type\":\"foundation.electrical.electrical\"}],\"Right\":[{\"id\":\"n\",\"label\":\"-\",\"type\":\"foundation.electrical.electrical\"}],\"Top\":[]}"
  Memristor11 : fl_lib/Electrical/Electrical Elements/Memristor  Ra=10500 Ohm  Rb=9500 Ohm  Q0=1.1e-2 C  x0=0.2  pwindow=2  i_specify=off  i_priority=None  i=0 A  i_nominal_specify=off  i_nominal_unit=A  i_nominal_value=1  v_specify=off  v_priority=None  v=0 V  v_nominal_specify=off  v_nominal_unit=V  v_nominal_value=1
      settings: InternalSimscapePortConfiguration="{\"Bottom\":[],\"Left\":[{\"id\":\"p\",\"label\":\"+\",\"type\":\"foundation.electrical.electrical\"}],\"Right\":[{\"id\":\"n\",\"label\":\"-\",\"type\":\"foundation.electrical.electrical\"}],\"Top\":[]}"
  Memristor12 : fl_lib/Electrical/Electrical Elements/Memristor  Ra=10500 Ohm  Rb=9500 Ohm  Q0=1.4e-2 C  x0=0.2  pwindow=2  i_specify=off  i_priority=None  i=0 A  i_nominal_specify=off  i_nominal_unit=A  i_nominal_value=1  v_specify=off  v_priority=None  v=0 V  v_nominal_specify=off  v_nominal_unit=V  v_nominal_value=1
      settings: InternalSimscapePortConfiguration="{\"Bottom\":[],\"Left\":[{\"id\":\"p\",\"label\":\"+\",\"type\":\"foundation.electrical.electrical\"}],\"Right\":[{\"id\":\"n\",\"label\":\"-\",\"type\":\"foundation.electrical.electrical\"}],\"Top\":[]}"
  Memristor13 : fl_lib/Electrical/Electrical Elements/Memristor  Ra=10500 Ohm  Rb=9500 Ohm  Q0=1.56e-2 C  x0=0.2  pwindow=2  i_specify=off  i_priority=None  i=0 A  i_nominal_specify=off  i_nominal_unit=A  i_nominal_value=1  v_specify=off  v_priority=None  v=0 V  v_nominal_specify=off  v_nominal_unit=V  v_nominal_value=1
      settings: InternalSimscapePortConfiguration="{\"Bottom\":[],\"Left\":[{\"id\":\"p\",\"label\":\"+\",\"type\":\"foundation.electrical.electrical\"}],\"Right\":[{\"id\":\"n\",\"label\":\"-\",\"type\":\"foundation.electrical.electrical\"}],\"Top\":[]}"
  Memristor14 : fl_lib/Electrical/Electrical Elements/Memristor  Ra=10500 Ohm  Rb=9500 Ohm  Q0=1.85e-2 C  x0=0.2  pwindow=2  i_specify=off  i_priority=None  i=0 A  i_nominal_specify=off  i_nominal_unit=A  i_nominal_value=1  v_specify=off  v_priority=None  v=0 V  v_nominal_specify=off  v_nominal_unit=V  v_nominal_value=1
      settings: InternalSimscapePortConfiguration="{\"Bottom\":[],\"Left\":[{\"id\":\"p\",\"label\":\"+\",\"type\":\"foundation.electrical.electrical\"}],\"Right\":[{\"id\":\"n\",\"label\":\"-\",\"type\":\"foundation.electrical.electrical\"}],\"Top\":[]}"
  Memristor15 : fl_lib/Electrical/Electrical Elements/Memristor  Ra=10500 Ohm  Rb=9500 Ohm  Q0=1.35e-2 C  x0=0.2  pwindow=2  i_specify=off  i_priority=None  i=0 A  i_nominal_specify=off  i_nominal_unit=A  i_nominal_value=1  v_specify=off  v_priority=None  v=0 V  v_nominal_specify=off  v_nominal_unit=V  v_nominal_value=1
      settings: InternalSimscapePortConfiguration="{\"Bottom\":[],\"Left\":[{\"id\":\"p\",\"label\":\"+\",\"type\":\"foundation.electrical.electrical\"}],\"Right\":[{\"id\":\"n\",\"label\":\"-\",\"type\":\"foundation.electrical.electrical\"}],\"Top\":[]}"
  Memristor16 : fl_lib/Electrical/Electrical Elements/Memristor  Ra=10500 Ohm  Rb=9500 Ohm  Q0=1.7e-2 C  x0=0.2  pwindow=2  i_specify=off  i_priority=None  i=0 A  i_nominal_specify=off  i_nominal_unit=A  i_nominal_value=1  v_specify=off  v_priority=None  v=0 V  v_nominal_specify=off  v_nominal_unit=V  v_nominal_value=1
      settings: InternalSimscapePortConfiguration="{\"Bottom\":[],\"Left\":[{\"id\":\"p\",\"label\":\"+\",\"type\":\"foundation.electrical.electrical\"}],\"Right\":[{\"id\":\"n\",\"label\":\"-\",\"type\":\"foundation.electrical.electrical\"}],\"Top\":[]}"
  Memristor9 : fl_lib/Electrical/Electrical Elements/Memristor  Ra=10500 Ohm  Rb=9500 Ohm  Q0=1.5e-2 C  x0=0.2  pwindow=2  i_specify=off  i_priority=None  i=0 A  i_nominal_specify=off  i_nominal_unit=A  i_nominal_value=1  v_specify=off  v_priority=None  v=0 V  v_nominal_specify=off  v_nominal_unit=V  v_nominal_value=1
      settings: InternalSimscapePortConfiguration="{\"Bottom\":[],\"Left\":[{\"id\":\"p\",\"label\":\"+\",\"type\":\"foundation.electrical.electrical\"}],\"Right\":[{\"id\":\"n\",\"label\":\"-\",\"type\":\"foundation.electrical.electrical\"}],\"Top\":[]}"
  Mux : Mux  Inputs=8
  PS-Simulink Converter{1..16} (16 alike) : nesl_utility/PS-Simulink Converter  PhysicalDomain=network_engine_domain  SubClassName=ps_output  LeftPortType=input  RightPortType=output  PseudoPeriodic=off  Frequencies=[]  VectorFormat=1-D array  Unit=inherit  AffineConversion=off
  Product{,1..7} (8 alike) : Product  Inputs=*/
  Simulink-PS Converter{,1..7} (8 alike) : nesl_utility/Simulink-PS Converter  PhysicalDomain=network_engine_domain  SubClassName=ps_input  LeftPortType=input  RightPortType=output  PseudoPeriodic=off  Frequencies=[]  NoiseDistribution=none  NoiseParameters=[]  Unit=1  AffineConversion=off  FilteringAndDerivatives=provide  SimscapeFilterOrder=1  InputFilterTimeConstant=0.001  UdotUserProvided=0
  Solver Configuration : nesl_utility/Solver Configuration  PhysicalDomain=network_engine_domain  SubClassName=solver  LeftPortType=input  RightPortType=generic  Tones=[]  Harmonics=[]  SimulateNoise=off  Profile=off  UseLocalSampling=off  EnableSwitchedLinearOptims=on  FrequencyDomain=off  UseCCode=off  RelTol=0.001  AbsTol=1e-06  MinStep=1e-09  ToWorkspace=off  RevertToSquareIcSolve=off  NumHomotopyIterations=100  PhasorMode=off  PhasorModeNumHarmonics=1  ConsistencySolver=NEWTON_XTOL_AFTER_FTOL  IndexReductionMethod=DerivativeReplacement  DoDC=off  ResidualTolerance=1e-09  ConsistencyTolSource=GLOBAL  ConsistencyAbsTol=0.001  ConsistencyRelTol=0.001  ConsistencyTolFactor=0.001  UseLocalSolver=on  LocalSolverChoice=NE_BACKWARD_EULER_ADVANCER  ResolveIndetEquations=on  FunctionEvalNumThread=1  LocalSolverSampleTime=0.001  DoFixedCost=on  MaxNonlinIter=3  MaxModeIter=2  ComputeImpulses=off  ImpulseIterations=2  LinearAlgebra=auto  LinearAlgebraNumThread=0  EquationFormulation=NE_TIME_EF  DelaysMemoryBudget=1024  AutomaticFiltering=on  FilteringTimeConstant=0.001  PartitionStorageMethod=AS_NEEDED  PartitionMemoryBudget=1024  PartitionMethod=ROBUST
  Voltage Sensor{1..7,9} (8 alike) : fl_lib/Electrical/Electrical Sensors/Voltage Sensor
  sens_next1 : Outport
  wires:
  PS-Simulink Converter11/1 -> Product5/1
  PS-Simulink Converter16/1 -> Product4/1
  PS-Simulink Converter7/1 -> Product5/2
  PS-Simulink Converter8/1 -> Product4/2
  PS-Simulink Converter15/1 -> Product6/1
  PS-Simulink Converter12/1 -> Product7/2
  PS-Simulink Converter13/1 -> Product6/2
  PS-Simulink Converter14/1 -> Product7/1
  PS-Simulink Converter5/1 -> Product3/1
  PS-Simulink Converter6/1 -> Product2/1
  PS-Simulink Converter3/1 -> Product3/2
  PS-Simulink Converter4/1 -> Product2/2
  PS-Simulink Converter2/1 -> Product1/1
  PS-Simulink Converter1/1 -> Product1/2
  PS-Simulink Converter10/1 -> Product/2
  PS-Simulink Converter9/1 -> Product/1
  Product7/1 -> Mux/8
  Product/1 -> Mux/1
  Product6/1 -> Mux/7
  Product2/1 -> Mux/3
  Product3/1 -> Mux/4
  Product1/1 -> Mux/2
  Product5/1 -> Mux/6
  Mux/1 -> sens_next1/1
  Product4/1 -> Mux/5
  Demux/1 -> Simulink-PS Converter/1
  Demux/4 -> Simulink-PS Converter3/1
  Demux/2 -> Simulink-PS Converter1/1
  Demux/6 -> Simulink-PS Converter5/1
  Demux/8 -> Simulink-PS Converter7/1
  Demux/7 -> Simulink-PS Converter6/1
  Demux/3 -> Simulink-PS Converter2/1
  drift_V/1 -> Demux/1
  Demux/5 -> Simulink-PS Converter4/1
  connections:
  Voltage Sensor6/RConn1 -- PS-Simulink Converter15/LConn1
  PS-Simulink Converter13/LConn1 -- Current Sensor6/RConn1
  PS-Simulink Converter7/LConn1 -- Current Sensor5/RConn1
  PS-Simulink Converter8/LConn1 -- Current Sensor4/RConn1
  Voltage Sensor4/RConn1 -- PS-Simulink Converter11/LConn1
  Current Sensor4/LConn1 -- Controlled Voltage Source5/LConn1
  Voltage Sensor7/RConn1 -- PS-Simulink Converter16/LConn1
  Voltage Sensor6/RConn2 -- Memristor15/RConn1 -- Voltage Sensor4/RConn2 -- Memristor13/RConn1 -- Voltage Sensor7/RConn2 -- Memristor16/RConn1 -- Voltage Sensor2/RConn2 -- Memristor11/RConn1 -- Voltage Sensor3/RConn2 -- Memristor12/RConn1 -- Voltage Sensor1/RConn2 -- Memristor10/RConn1 -- Voltage Sensor9/RConn2 -- Memristor9/RConn1 -- Electrical Reference1/LConn1 -- Memristor14/RConn1 -- Voltage Sensor5/RConn2
  Controlled Voltage Source7/LConn1 -- Current Sensor6/LConn1
  Current Sensor5/LConn1 -- Controlled Voltage Source6/LConn1
  Voltage Sensor5/RConn1 -- PS-Simulink Converter14/LConn1
  Current Sensor7/LConn1 -- Controlled Voltage Source8/LConn1
  PS-Simulink Converter12/LConn1 -- Current Sensor7/RConn1
  Voltage Sensor4/LConn1 -- Memristor13/LConn1 -- Current Sensor5/RConn2
  Voltage Sensor7/LConn1 -- Memristor16/LConn1 -- Current Sensor4/RConn2
  Voltage Sensor5/LConn1 -- Memristor14/LConn1 -- Current Sensor7/RConn2
  Voltage Sensor6/LConn1 -- Memristor15/LConn1 -- Current Sensor6/RConn2
  Voltage Sensor3/RConn1 -- PS-Simulink Converter6/LConn1
  PS-Simulink Converter4/LConn1 -- Current Sensor2/RConn1
  PS-Simulink Converter3/LConn1 -- Current Sensor3/RConn1
  Controlled Voltage Source3/LConn1 -- Current Sensor2/LConn1
  Voltage Sensor2/RConn1 -- PS-Simulink Converter5/LConn1
  Controlled Voltage Source4/LConn1 -- Current Sensor3/LConn1
  Voltage Sensor2/LConn1 -- Memristor11/LConn1 -- Current Sensor3/RConn2
  Voltage Sensor3/LConn1 -- Memristor12/LConn1 -- Current Sensor2/RConn2
  PS-Simulink Converter1/LConn1 -- Current Sensor1/RConn1
  Voltage Sensor1/RConn1 -- PS-Simulink Converter2/LConn1
  Controlled Voltage Source2/LConn1 -- Current Sensor1/LConn1
  Voltage Sensor1/LConn1 -- Memristor10/LConn1 -- Current Sensor1/RConn2
  Simulink-PS Converter1/RConn1 -- Controlled Voltage Source2/RConn1
  Current Sensor/LConn1 -- Controlled Voltage Source1/LConn1
  PS-Simulink Converter10/LConn1 -- Current Sensor/RConn1
  Voltage Sensor9/RConn1 -- PS-Simulink Converter9/LConn1
  Current Sensor/RConn2 -- Voltage Sensor9/LConn1 -- Memristor9/LConn1
  Simulink-PS Converter6/RConn1 -- Controlled Voltage Source7/RConn1
  Controlled Voltage Source3/RConn1 -- Simulink-PS Converter2/RConn1
  Controlled Voltage Source6/RConn1 -- Simulink-PS Converter5/RConn1
  Controlled Voltage Source4/RConn1 -- Simulink-PS Converter3/RConn1
  Controlled Voltage Source8/RConn1 -- Simulink-PS Converter7/RConn1
  Controlled Voltage Source1/RConn1 -- Simulink-PS Converter/RConn1
  Controlled Voltage Source5/RConn1 -- Simulink-PS Converter4/RConn1
  Electrical Reference2/LConn1 -- Solver Configuration/RConn1 -- Controlled Voltage Source8/RConn2 -- Controlled Voltage Source7/RConn2 -- Controlled Voltage Source6/RConn2 -- Controlled Voltage Source5/RConn2 -- Controlled Voltage Source4/RConn2 -- Controlled Voltage Source3/RConn2 -- Controlled Voltage Source2/RConn2 -- Controlled Voltage Source1/RConn2
